simulink model "ensaio"  (R2023b)
settings: Solver=ode4  StartTime=0.0  StopTime=80  FixedStep=0.001  RelTol=1e-3
undefined symbols (not defined in the file or in its folder): sigbuilder_block
libraries: simulink_extras x2
settings Model: SimulationMode=accelerator  Creator=colom  LastModifiedBy=Paulo
settings SolverCC: AlgebraicLoopSolver=TrustRegion  AutoInsertRateTranBlk=on
settings OptimizationCC: LifeSpan=inf
settings DebuggingCC: SFExecutionAtInitializationDiag=none  ArithmeticOperatorsInVariantConditions=warning
settings HardwareCC: ProdBitPerSizeT=32  ProdBitPerPtrDiffT=32  ProdWordSize=32  ProdHWDeviceType=Specified
settings ModelReferenceCC: EnableRefExpFcnMdlSchedulingChecks=on
settings SFSimCC: CustomCodeUndefinedFunction=UseInterfaceOnly
settings CodeAppCC: StateflowObjectComments=on

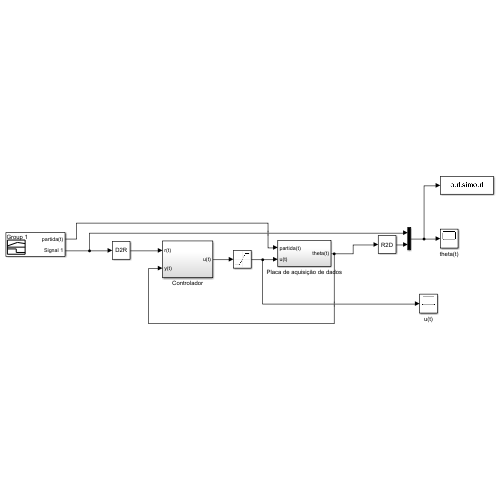
[thumbnail: Simulink's stored preview of the top-level diagram]
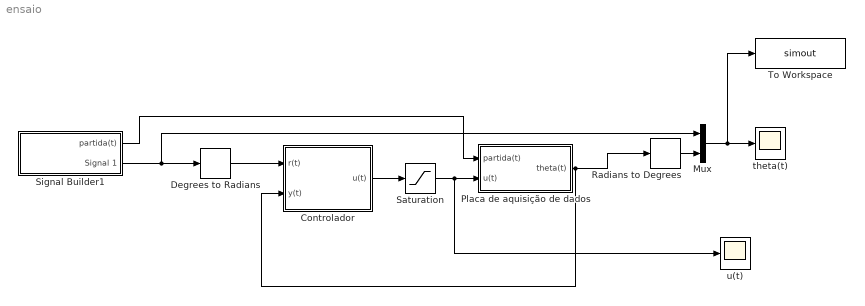
== system ensaio ==
  Controlador : Subsystem
  Degrees to Radians : simulink_extras/Transformations/Degrees to Radians
  Mux : Mux  Inputs=2
  Placa de aquisição de dados : Subsystem
  Radians to Degrees : simulink_extras/Transformations/Radians to Degrees
  Saturation : Saturate  UpperLimit=100  LowerLimit=0
  Signal Builder1 : Subsystem  Tag=STV Subsys  LoadFcn=sigbuilder_block('load');  StartFcn=sigbuilder_block('start');  StopFcn=sigbuilder_block('stop');  ClipboardFcn=sigbuilder_block('clipboard');  mask(Sigbuilder block){tuvar=[0:10]}
      mask help: Simulink:masks:SigbuilderBlock_MD
      mask init:
      | if ~strcmp(get_param(bdroot(gcbh),'SimulationStatus'),'stopped') tuvar = sigbuilder_block('maskInit'); end
      settings: CopyFcn=sigbuilder_block('copy');  DeleteFcn=sigbuilder_block('delete');  ModelCloseFcn=sigbuilder_block('modelClose');  PreSaveFcn=sigbuilder_block('preSave');  PauseFcn=sigbuilder_block('pause');  ContinueFcn=sigbuilder_block('continue');  NameChangeFcn=sigbuilder_block('namechange');  OpenFcn=sigbuilder_block('open',[5.4 36 1141.2 516.6 ]);  CloseFcn=sigbuilder_block('close');
      mask Display: plot(0, 0, 100, 100,[2, 2, 32, 32, 2], [68, 8, 8, 68, 68],[32, 2], [38, 38], [32, 19, 2],[53, 60, 44], [32, 17, 17, 2],[16, 16, 31, 31]);txt = getActiveGroup(gcbh);text(2, 100, txt,'verticalAlignment', 'top');
  To Workspace : ToWorkspace  VariableName=simout  SaveFormat=Timeseries  SampleTime=-1
  theta(t) : Scope
  u(t) : Scope
  wires:
  Signal Builder1/1(partida(t)) -> Placa de aquisição de dados/1(partida(t))
  Saturation/1 -> Placa de aquisição de dados/2(u(t)), u(t)/1
  Signal Builder1/2(Signal 1) -> Mux/1, Degrees to Radians/1
  Placa de aquisição de dados/1(theta(t)) -> Controlador/2(y(t)), Radians to Degrees/1
  Mux/1 -> To Workspace/1, theta(t)/1
  Radians to Degrees/1 -> Mux/2
  Degrees to Radians/1 -> Controlador/1(r(t))
  Controlador/1(u(t)) -> Saturation/1

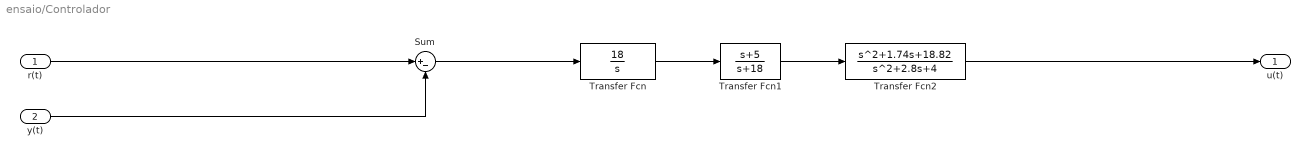
== system ensaio/Controlador ==
  r(t) : Inport
  y(t) : Inport  Port=2
  Sum : Sum  Inputs=|+-
  Transfer Fcn : TransferFcn  Numerator=[18]  Denominator=[1 0]
  Transfer Fcn1 : TransferFcn  Numerator=[1 5]  Denominator=[1 18]
  Transfer Fcn2 : TransferFcn  Numerator=[1 1.74 18.82]  Denominator=[1 2.8 4]
  u(t) : Outport  VectorParamsAs1DForOutWhenUnconnected=off
  wires:
  y(t)/1 -> Sum/2
  Transfer Fcn2/1 -> u(t)/1
  r(t)/1 -> Sum/1
  Transfer Fcn/1 -> Transfer Fcn1/1
  Transfer Fcn1/1 -> Transfer Fcn2/1
  Sum/1 -> Transfer Fcn/1

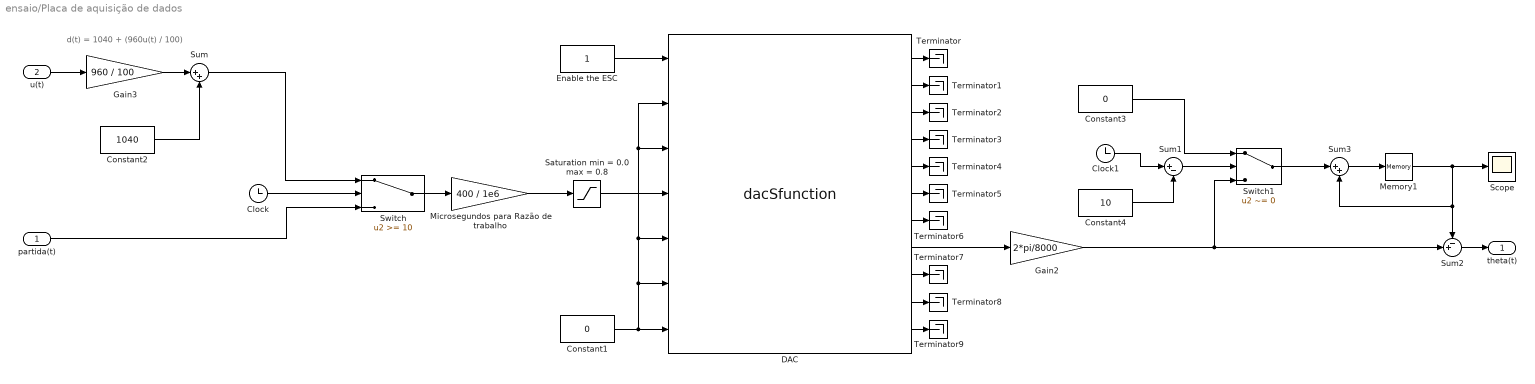
== system ensaio/Placa de aquisição de dados ==
  note: d(t) = 1040 + (960u(t) / 100)
  partida(t) : Inport
  u(t) : Inport  Port=2
  Clock : Clock
  Clock1 : Clock
  Constant1 : Constant  Value=0
  Constant2 : Constant  Value=1040
  Constant3 : Constant  Value=0
  Constant4 : Constant  Value=10
  DAC : S-Function  FunctionName=dacSfunction  Parameters=serialPort,sampleTime,gpioOutCh1FinalState,gpioOutCh2FinalState,gpioOutCh3FinalState,pwmFrequency,pwmCh1FinalDuty,pwmCh2FinalDuty,pwmCh3FinalDuty,pwmCh4FinalDuty,enc1Mode,enc1ResetCount,enc1Direction,enc1Quadrature,enc1Filter,enc2Mode,enc2ResetCount,enc2Direction,enc2Quadrature,enc2Filter,enc3Mode,enc3ResetCount,enc3Direction,enc3Quadrature,enc3Filter  SFunctionDeploymentMode=off  EnableBusSupport=off  mask{serialPort='COM3', sampleTime=10, gpioOutCh1FinalState=Low, gpioOutCh2FinalState=Low, gpioOutCh3FinalState=Low, pwmFrequency=400, pwmCh1FinalDuty=0, pwmCh2FinalDuty=0, pwmCh3FinalDuty=0, pwmCh4FinalDuty=0, enc1Mode=Counter, enc1Direction=Counter Clock Wise is positive, enc1Quadrature=High resolution, enc1Filter=15, enc1ResetCount=on, enc2Mode=Counter, enc2Direction=Counter Clock Wise is positive, enc2Quadrature=High resolution, enc2Filter=15, enc2ResetCount=off, enc3Mode=Counter, enc3Direction=Clock Wise is positive, enc3Quadrature=High resolution, enc3Filter=15, enc3ResetCount=off}
      mask prompts: serialPort "Serial port"; sampleTime "Sample time (ms)"; gpioOutCh1FinalState "Final state"; gpioOutCh2FinalState "Final state"; gpioOutCh3FinalState "Final state"; pwmFrequency "Frequency (Hz)"; pwmCh1FinalDuty "Final duty"; pwmCh2FinalDuty "Final duty"; pwmCh3FinalDuty "Final duty"; pwmCh4FinalDuty "Final duty"; enc1Mode "Mode"; enc1Direction "Direction"; enc1Quadrature "Resolution"; enc1Filter "Filter"; enc1ResetCount "Reset count"; enc2Mode "Mode"; enc2Direction "Direction"; enc2Quadrature "Resolution"; enc2Filter "Filter"; enc2ResetCount "Reset count"; enc3Mode "Mode"; enc3Direction "Direction"; enc3Quadrature "Resolution"; enc3Filter "Filter"; enc3ResetCount "Reset count"
      mask init:
      | % The first list item is initiated with 1 and not 0
      mask TypeOptions gpioOutCh1FinalState: Low | High
      mask TypeOptions gpioOutCh2FinalState: Low | High
      mask TypeOptions gpioOutCh3FinalState: Low | High
      mask TypeOptions enc1Mode: Counter | Time measurement
      mask TypeOptions enc1Direction: Counter Clock Wise is positive | Clock Wise is positive
      mask TypeOptions enc1Quadrature: Low resolution | High resolution
      mask TypeOptions enc2Mode: Counter | Time measurement
      mask TypeOptions enc2Direction: Counter Clock Wise is positive | Clock Wise is positive
      mask TypeOptions enc2Quadrature: Low resolution | High resolution
      mask TypeOptions enc3Mode: Counter | Time measurement
      mask TypeOptions enc3Direction: Counter Clock Wise is positive | Clock Wise is positive
      mask TypeOptions enc3Quadrature: Low resolution | High resolution
      mask DialogControl DescTextVar Prompt: %<MaskDescription> OpenDAC configuration
      mask DialogControl Container18 Prompt: General configuration
      mask DialogControl Container8 Prompt: GPIO Output
      mask DialogControl Container19 Prompt: Channel 1
      mask DialogControl Container22 Prompt: Channel 2
      mask DialogControl Container21 Prompt: Channel 3
      mask DialogControl Container6 Prompt: PWM
      mask DialogControl Container42 Prompt: General
      mask DialogControl Container43 Prompt: Channel 1
      mask DialogControl Container11 Prompt: Channel 2
      mask DialogControl Container12 Prompt: Channel 3
      mask DialogControl Container13 Prompt: Channel 4
      mask DialogControl Container4 Prompt: Encoders
      mask DialogControl Container35 Prompt: Encoder 1
      mask DialogControl Container36_copy Prompt: Encoder 2
      mask DialogControl Container36 Prompt: Encoder 3
      mask Display:
      | % Give names to the input ports
      | port_label('input', 1, 'Digital Out CH1 (PC15)');
      | port_label('input', 2, 'Digital Out CH2 (PC14)');
      | port_label('input', 3, 'Digital Out CH3 (PC13)');
      | port_label('input', 4, 'PWM CH1 (PB6)');
      | port_label('input', 5, 'PWM CH2 (PB7)');
      | port_label('input', 6, 'PWM CH3 (PB8)');
      | port_label('input', 7, 'PWM CH4 (PB9)');
      | 
      | % Give names to the output ports
      | port_label('output', 1, 'Digital In CH1 (PB12)');
      | port_label('output', 2, 'Digital In CH2 (PB13)');
      | port_label('output', 3, 'Digital In CH3 (PB14)');
      | port_label('output', 4, 'Analog In CH1 (PA0)');
      | port_label('output', 5, 'Analog In CH2 (PA1)');
      | port_label('output', 6, 'Analog In CH3 (PA4)');
      | port_label('output', 7, 'Analog In CH4 (PB0)');
      | port_label('output', 8, 'Encoder 1 (PA8/PA9)');
      | port_label('output', 9, 'Encoder 2 (PA15/PB3)');
      | port_label('output', 10, 'Encoder 3 (PB4/PB5)');
      | port_label('output', 11, 'Real Time Clock');
  Enable the ESC : Constant
  Gain2 : Gain  Gain=2*pi/8000
  Gain3 : Gain  Gain=960 / 100
  Memory1 : Memory
  Microsegundos para Razão de trabalho : Gain  Gain=400 / 1e6
  Saturation min = 0.0 max = 0.8 : Saturate  UpperLimit=0.8  LowerLimit=0.0
  Scope : Scope
  Sum : Sum  Inputs=|++
  Sum1 : Sum  Inputs=|+-
  Sum2 : Sum  Inputs=-+|
  Sum3 : Sum  Inputs=|++
  Switch : Switch  Threshold=10  SaturateOnIntegerOverflow=off  InputSameDT=off
  Switch1 : Switch  Criteria=u2 ~= 0  SaturateOnIntegerOverflow=off  InputSameDT=off
  Terminator{,1..9} (10 alike) : Terminator
  theta(t) : Outport  VectorParamsAs1DForOutWhenUnconnected=off
  wires:
  DAC/8 -> Gain2/1
  Constant1/1 -> DAC/3, DAC/2, DAC/5, DAC/6, DAC/7
  Enable the ESC/1 -> DAC/1
  Gain2/1 -> Switch1/3, Sum2/2
  Gain3/1 -> Sum/1
  Constant2/1 -> Sum/2
  DAC/2 -> Terminator1/1
  DAC/1 -> Terminator/1
  DAC/3 -> Terminator2/1
  DAC/4 -> Terminator3/1
  DAC/5 -> Terminator4/1
  DAC/6 -> Terminator5/1
  DAC/7 -> Terminator6/1
  DAC/9 -> Terminator7/1
  DAC/10 -> Terminator8/1
  DAC/11 -> Terminator9/1
  Saturation min = 0.0 max = 0.8/1 -> DAC/4
  u(t)/1 -> Gain3/1
  Microsegundos para Razão de trabalho/1 -> Saturation min = 0.0 max = 0.8/1
  Switch/1 -> Microsegundos para Razão de trabalho/1
  Clock/1 -> Switch/2
  Sum/1 -> Switch/1
  partida(t)/1 -> Switch/3
  Sum2/1 -> theta(t)/1
  Memory1/1 -> Sum3/2, Sum2/1, Scope/1
  Switch1/1 -> Sum3/1
  Sum3/1 -> Memory1/1
  Constant3/1 -> Switch1/1
  Clock1/1 -> Sum1/1
  Constant4/1 -> Sum1/2
  Sum1/1 -> Switch1/2

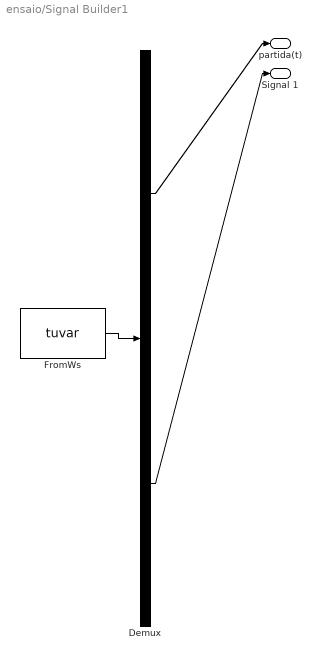
== system ensaio/Signal Builder1 ==
  Demux : Demux  Tag=STV Demux  Outputs=2
      settings: DisplayOption=none
  FromWs : FromWorkspace  Tag=STV FromWs  VariableName=tuvar
      SigBuilderData=|
      | common.afterFinalStr = 'Extrapolate'
      | common.sampleTime = 0
      | dataSet.timeRange = [0 80]
      | dataSet.name = 'Group 1'
      | sbobj.Groups.Name = 'Group 1'
      | sbobj.Groups.Signals(1).Name = 'partida(t)'
      | sbobj.Groups.Signals(1).XData = [0 0.5 0.5 2.5 2.5 6.5 6.5 10 10 15 16 17 18 19 80]
      | sbobj.Groups.Signals(1).YData = [0 0 2000 2000 2 0 1040 1040 4 0 0 0 0 0 0]
      | sbobj.Groups.Signals(2).Name = 'Signal 1'
      | sbobj.Groups.Signals(2).XData = [0 10 15 20 30 30 36 39 47 52 72 73 74 75 76 77 78 79 80]
      | sbobj.Groups.Signals(2).YData = [0 0 15 30 30 35 35 35 35 35 0 0 0 0 0 0 0 0 0]
      | sbobj.Groups.TimeRange = [0 80]
  partida(t) : Outport  Tag=STV Outport  VectorParamsAs1DForOutWhenUnconnected=off
  Signal 1 : Outport  Tag=STV Outport  Port=2  VectorParamsAs1DForOutWhenUnconnected=off
  wires:
  FromWs/1 -> Demux/1
  Demux/1 -> partida(t)/1
  Demux/2 -> Signal 1/1
